simulink model "switch_control"  (Simulink 6.3)
settings: Solver=FixedStepDiscrete  StartTime=0.0  StopTime=10.0  RelTol=1e-3
InitFcn:
  | %% DSPBuilder Start
  | alt_dspbuilder_update_model(bdroot)
  | %% DSPBuilder End
libraries: allblocks_alteradspbuilder2 x8
settings Model: Creator=gnixon  LastModifiedBy=gnixon
settings OptimizationCC: BlockReduction=off  BooleanDataType=off  InlineInvariantSignals=on
settings DebuggingCC: SolverPrmCheckMsg=none
settings HardwareCC: TargetUnknown=on

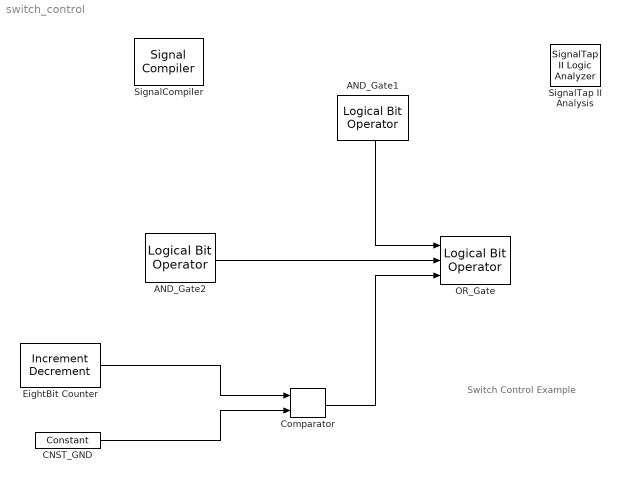
== system switch_control ==
  note: Switch Control Example
  AND_Gate1 : allblocks_alteradspbuilder2/Logical Bit Operator  Orientation=down  LogicalOperator=AND  user_inputs=2
  AND_Gate2 : allblocks_alteradspbuilder2/Logical Bit Operator  LogicalOperator=AND  user_inputs=2
  CNST_GND : allblocks_alteradspbuilder2/Constant  mask_cst=0  BusType=Unsigned Integer  bwl=8  bwr=0  UseDefaultClock=on
  Comparator : allblocks_alteradspbuilder2/Comparator  direction=a == b
  EightBit Counter : allblocks_alteradspbuilder2/Increment Decrement  BusType=Unsigned Integer  bwl=8  bwr=0  UseDefaultClock=on  clr_value=0  direction=Increment  phase_selection=1  use_ena=off  use_sclr=off
  OR_Gate : allblocks_alteradspbuilder2/Logical Bit Operator  LogicalOperator=OR  user_inputs=3
  SignalCompiler : allblocks_alteradspbuilder2/Signal Compiler  DeviceFamily=DSP Board  DeviceName=AUTO  EnableSignalTap=on  SignalTapDepth=128  UseBoardBlock=off  StpUseDefaultClock=on  StpClock=clock
  SignalTap II Analysis : allblocks_alteradspbuilder2/SignalTap II Logic Analyzer
  wires:
  EightBit Counter/1 -> Comparator/1
  CNST_GND/1 -> Comparator/2
  AND_Gate2/1 -> OR_Gate/2
  Comparator/1 -> OR_Gate/3
  AND_Gate1/1 -> OR_Gate/1
